simulink model "smm_simple_2015a"  (R2015a)
settings: Solver=ode45  StartTime=0.0  StopTime=50  MaxStep=1e-3  RelTol=1e-4  AbsTol=1e-6
InitFcn:
  | rng shuffle
values from neighbouring files (symbols this model uses):
  a0 = 68*pi/180    (= 1.18682389136)    [smm_params_simple.m]
  dx0 = 5    [smm_params_simple.m]
  dy0 = 0    [smm_params_simple.m]
  g = 9.81    [smm_params_simple.m]
  k = 20000    [smm_params_simple.m]
  l0 = 1    [smm_params_simple.m]
  m = 80    [smm_params_simple.m]
  x0 = 0    [smm_params_simple.m]
  y0 = l0    (= 1)    [smm_params_simple.m]
libraries: simulink_extras x1
settings Model: Creator=hgeyer  LastModifiedBy=Joe
settings DataIOCC: SignalLoggingSaveFormat=ModelDataLogs
settings OptimizationCC: ExpressionDepthLimit=2147483647
settings DebuggingCC: UnderspecifiedInitializationDetection=Classic  MergeDetectMultiDrivingBlocksExec=none  SolverPrmCheckMsg=warning  FcnCallInpInsideContextMsg=EnableAllAsWarning  StateNameClashWarn=warning

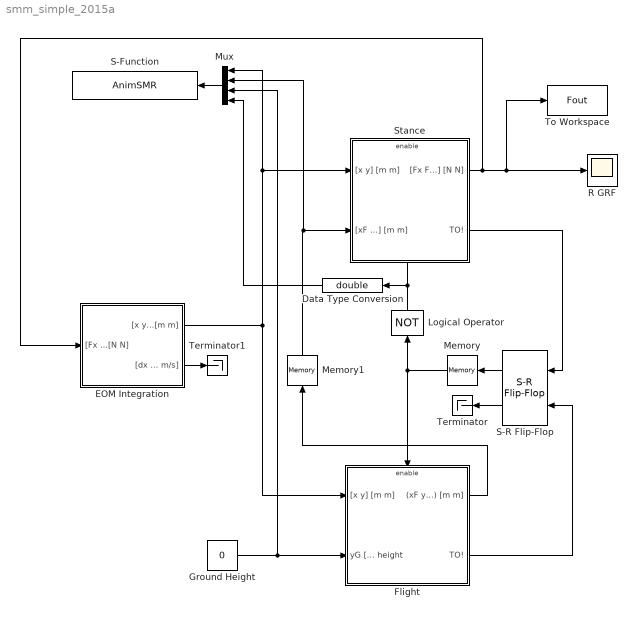
== system smm_simple_2015a ==
  Data Type Conversion : DataTypeConversion  OutDataTypeStr=double
  EOM Integration : Subsystem
  Flight : Subsystem
  Ground Height : Constant  Value=0
  Logical Operator : Logic  Operator=NOT  AllPortsSameDT=off  OutDataTypeStr=boolean
  Memory : Memory  X0=1
  Memory1 : Memory  X0=[0 0]
  Mux : Mux
  R GRF : Scope
      settings: TimeRange=auto  LimitDataPoints=on  MaxDataPoints=5000  SaveToWorkspace=off  SaveName=ScopeData  YMin=-10  YMax=10  SampleTime=-1
  S-Function : S-Function  FunctionName=AnimSMR  Parameters=0.01  SFunctionDeploymentMode=off  EnableBusSupport=off
  S-R Flip-Flop : simulink_extras/Flip Flops/S-R Flip-Flop  initial_condition=1
  Stance : Subsystem
  Terminator : Terminator
  Terminator1 : Terminator
  To Workspace : ToWorkspace  VariableName=Fout  SaveFormat=Timeseries  SampleTime=-1
      settings: MaxDataPoints=1
  wires:
  EOM Integration/1("[x y] [m m]") -> Stance/1("[x y] [m m]"), Mux/1, Flight/1("[x y] [m m]")
  Stance/2(TO!) -> S-R Flip-Flop/1
  S-R Flip-Flop/1 -> Memory/1
  Logical Operator/1 -> Stance/Enable, Data Type Conversion/1
  Memory/1 -> Logical Operator/1, Flight/Enable
  Flight/2(TO!) -> S-R Flip-Flop/2
  Stance/1("[Fx Fy] [N N]") -> EOM Integration/1("[Fx Fy] [N N]"), To Workspace/1, R GRF/1
  Flight/1((xF yF) [m m]) -> Memory1/1
  Memory1/1 -> Mux/2, Stance/2("[xF yF] [m m]")
  Mux/1 -> S-Function/1
  S-R Flip-Flop/2 -> Terminator/1
  Ground Height/1 -> Mux/3, Flight/2(yG [m] ground height)
  Data Type Conversion/1 -> Mux/4
  EOM Integration/2("[dx dy] [m/s m/s]") -> Terminator1/1

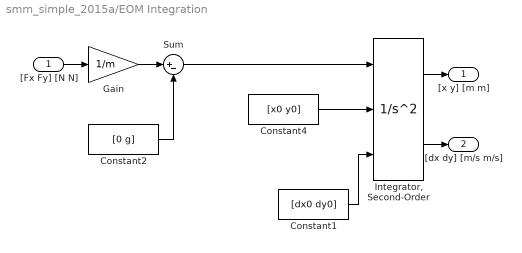
== system smm_simple_2015a/EOM Integration ==
  "[Fx Fy] [N N]" : Inport
  Constant1 : Constant  Value=[dx0 dy0]
  Constant2 : Constant  Value=[0 g]
  Constant4 : Constant  Value=[x0 y0]
  Gain : Gain  Gain=1/m
  "Integrator, Second-Order" : SecondOrderIntegrator  ICSourceX=external  ICSourceDXDT=external
  Sum : Sum  Inputs=|+-
  "[x y] [m m]" : Outport
  "[dx dy] [m/s m/s]" : Outport  Port=2
  wires:
  Constant1/1 -> "Integrator, Second-Order"/3
  Gain/1 -> Sum/1
  Sum/1 -> "Integrator, Second-Order"/1
  Constant2/1 -> Sum/2
  "[Fx Fy] [N N]"/1 -> Gain/1
  "Integrator, Second-Order"/1 -> "[x y] [m m]"/1
  "Integrator, Second-Order"/2 -> "[dx dy] [m/s m/s]"/1
  Constant4/1 -> "Integrator, Second-Order"/2

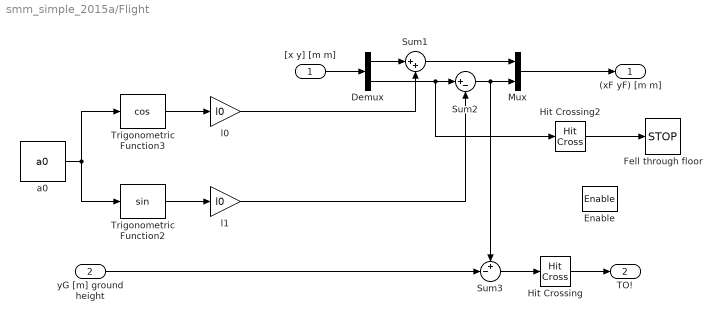
== system smm_simple_2015a/Flight ==
  "[x y] [m m]" : Inport
  yG [m] ground height : Inport  Port=2
  Enable : EnablePort  StatesWhenEnabling=reset
  Demux : Demux  Outputs=2
  Fell through floor : Stop
  Hit Crossing : HitCross  HitCrossingDirection=falling
  Hit Crossing2 : HitCross  HitCrossingDirection=falling
  Mux : Mux  Inputs=2
  Sum1 : Sum  Inputs=|++
  Sum2 : Sum  Inputs=|+-
  Sum3 : Sum  Inputs=+-|
  Trigonometric Function2 : Trigonometry
  Trigonometric Function3 : Trigonometry  Operator=cos
  a0 : Constant  Value=a0
  l0 : Gain  Gain=l0
  l1 : Gain  Gain=l0
  (xF yF) [m m] : Outport  InitialOutput=0
      settings: AttributesFormatString=%<OutputWhenDisabled>
  TO! : Outport  Port=2  OutputWhenDisabled=reset  InitialOutput=0
  wires:
  Hit Crossing/1 -> TO!/1
  a0/1 -> Trigonometric Function3/1, Trigonometric Function2/1
  Trigonometric Function3/1 -> l0/1
  Trigonometric Function2/1 -> l1/1
  "[x y] [m m]"/1 -> Demux/1
  Demux/1 -> Sum1/1
  l0/1 -> Sum1/2
  l1/1 -> Sum2/2
  Demux/2 -> Hit Crossing2/1, Sum2/1
  Sum1/1 -> Mux/1
  Sum2/1 -> Mux/2, Sum3/1
  Mux/1 -> (xF yF) [m m]/1
  yG [m] ground height/1 -> Sum3/2
  Sum3/1 -> Hit Crossing/1
  Hit Crossing2/1 -> Fell through floor/1

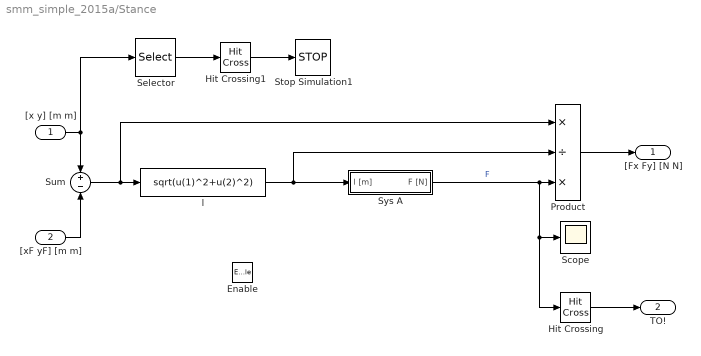
== system smm_simple_2015a/Stance ==
  "[x y] [m m]" : Inport
  "[xF yF] [m m]" : Inport  Port=2
  Enable : EnablePort  StatesWhenEnabling=reset
  Hit Crossing : HitCross  HitCrossingDirection=falling
  Hit Crossing1 : HitCross  HitCrossingDirection=falling
  Product : Product  Inputs=*/*  RndMeth=Zero
  Scope : Scope
      settings: TimeRange=auto  MaxDataPoints=5000  SaveToWorkspace=off  YMin=-213.40424  YMax=1934.05985  SampleTime=-1
  Selector : Selector  InputPortWidth=2  IndexOptions=Index vector (dialog)  Indices=[2]  OutputSizes=1
  Stop Simulation1 : Stop
  Sum : Sum  Inputs=+-
  Sys A : Subsystem
  l : Fcn  Expr=sqrt(u(1)^2+u(2)^2)
  "[Fx Fy] [N N]" : Outport  OutputWhenDisabled=reset  InitialOutput=[0 0]
      settings: AttributesFormatString="when disabled: \"%<OutputWhenDisabled>\""
  TO! : Outport  Port=2  OutputWhenDisabled=reset  InitialOutput=[0]
      settings: AttributesFormatString="when disabled: \"%<OutputWhenDisabled>\""
  wires:
  Product/1 -> "[Fx Fy] [N N]"/1
  "[xF yF] [m m]"/1 -> Sum/2
  "[x y] [m m]"/1 -> Selector/1, Sum/1
  Sum/1 -> Product/1, l/1
  Hit Crossing/1 -> TO!/1
  l/1 -> Product/2, Sys A/1(l [m])
  Sys A/1(F [N]) -> Hit Crossing/1, Scope/1, Product/3  "F"
  Selector/1 -> Hit Crossing1/1
  Hit Crossing1/1 -> Stop Simulation1/1

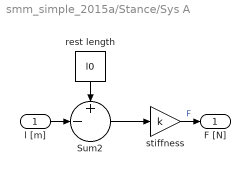
== system smm_simple_2015a/Stance/Sys A ==
  l [m] : Inport
  Sum2 : Sum  Inputs=+-|
  rest length : Constant  Value=l0
  stiffness : Gain  Gain=k
  F [N] : Outport
  wires:
  l [m]/1 -> Sum2/2
  stiffness/1 -> F [N]/1  "F"
  Sum2/1 -> stiffness/1
  rest length/1 -> Sum2/1
